simulink model "DC_grid_simple"  (R2018a)
settings: Solver=VariableStepAuto  StartTime=0.0  StopTime=10  RelTol=1e-3
values from neighbouring files (symbols this model uses):
  inputsFromWS = Simulink.Parameter(inputArray)    [DC_grid.m]    (also in QlearningEMS.m; QlearningEMS_Average.m; init_for_DC_grid.m)
libraries: SignalEditorBlockLib x1, powerlib x1
settings Model: SimulationMode=accelerator  Creator=David Pasdeloup  LastModifiedBy=David Pasdeloup
settings DataIOCC: FinalStateName=myOperPoint  LoadInitialState=on  SaveFinalState=on  SaveCompleteFinalSimState=on
settings DebuggingCC: MaxConsecutiveZCsMsg=none

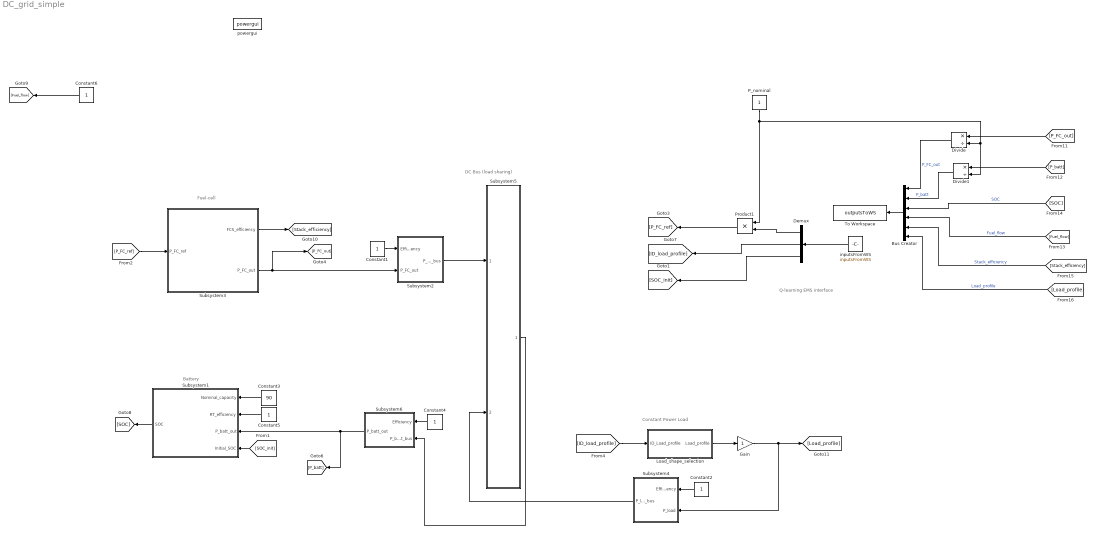
== system DC_grid_simple ==
  note: DC Bus (load sharing)
  note: Q-learning EMS interface
  note: Fuel-cell
  note: Battery
  note: Constant Power Load
  Bus Creator : BusCreator  Inputs=6
  Constant{1..2,4..6} (5 alike) : Constant
  Constant3 : Constant  Value=90
  Demux : Demux  Outputs=3
  Divide : Product  Inputs=*/
  Divide1 : Product  Inputs=*/
  Gain : Gain
  Load_shape_selection : Subsystem
  P_nominal : Constant
  Product1 : Product
  Subsystem1 : Subsystem
  Subsystem2 : Subsystem
  Subsystem3 : Subsystem
  Subsystem4 : Subsystem
  Subsystem5 : Subsystem
  Subsystem6 : Subsystem
  To Workspace : ToWorkspace  VariableName=outputsToWS  SaveFormat=Timeseries  SampleTime=-1
  inputsFromWS : Constant  Value=inputsFromWS
  powergui : powerlib/powergui  SimulationMode=Continuous  SampleTime=1e-6  frequency=60  Iterations=50  frequencyindice=0  Pbase=100e6  ErrMax=1e-4  UnitsV=kV  UnitsW=MW  buscounter=0  FunctionMessages=off  echomessages=off  EnableUseOfTLC=off  CurrentSourceSwitches=off  DisableSnubberDevices=off  DisableRonSwitches=off  DisableVfSwitches=off  DisplayEquations=off  SolverType=Tustin/Backward Euler (TBE)  Interpol=off  ExternalGateDelay=off  methode=off  Ts=100  x0status=blocks  SPID=on  SwTol=0  HookPort=off  RestoreLinks=warning  ResistiveCurrentMeasurement=off  Frange=[0:2:500]  Ylog=off  Xlog=on  ShowGrid=off  save=off  variable=ZData  structure=0  ZoomFFT=on  StartTime=0.0  cycles=1  DisplayStyle=1  fundamental=60  FreqAxis=off  MaxFrequency=1000  frequencyindicesteady=1  RmsSteady=1  display=off
  wires:
  Demux/1 -> Product1/2
  Demux/2 -> [ID_load_profile]
  Bus Creator/1 -> To Workspace/1
  [P_batt] -> Divide1/1
  Divide1/1 -> Bus Creator/2  "P_batt"
  inputsFromWS/1 -> Demux/1
  Product1/1 -> [P_FC_ref]
  Divide/1 -> Bus Creator/1  "P_FC_out"
  P_nominal/1 -> Divide1/2, Divide/2, Product1/1
  [P_FC_out] -> Divide/1
  [SOC] -> Bus Creator/3  "SOC"
  [Fuel_flow] -> Bus Creator/4  "Fuel_flow"
  [Stack_efficiency] -> Bus Creator/5  "Stack_efficiency"
  [ID_load_profile] -> Load_shape_selection/1(ID_Load_profile)
  Load_shape_selection/1(Load_profile) -> Gain/1
  [Load_profile] -> Bus Creator/6  "Load_profile"
  Demux/3 -> [SOC_init]
  Subsystem6/1(P_batt_out) -> [P_batt], Subsystem1/3(P_batt_out)
  Constant4/1 -> Subsystem6/1(Efficiency)
  Constant3/1 -> Subsystem1/1(Nominal_capacity)
  Constant5/1 -> Subsystem1/2(RT_efficiency)
  [SOC_init] -> Subsystem1/4(Initial_SOC)
  Subsystem1/1(SOC) -> [SOC]
  Constant1/1 -> Subsystem2/1(Efficiency)
  Subsystem3/2(P_FC_out) -> [P_FC_out], Subsystem2/2(P_FC_out)
  [P_FC_ref] -> Subsystem3/1(P_FC_ref)
  Subsystem3/1(FCS_efficiency) -> [Stack_efficiency]
  Constant2/1 -> Subsystem4/1(Efficiency)
  Subsystem2/1(P_FC_bus) -> Subsystem5/1(P_FC_bus)
  Subsystem4/1(P_load_bus) -> Subsystem5/2(P_load_bus)
  Subsystem5/1(P_batt_bus) -> Subsystem6/2(P_batt_bus)
  Constant6/1 -> [Fuel_flow]
  Gain/1 -> Subsystem4/2(P_load), [Load_profile]

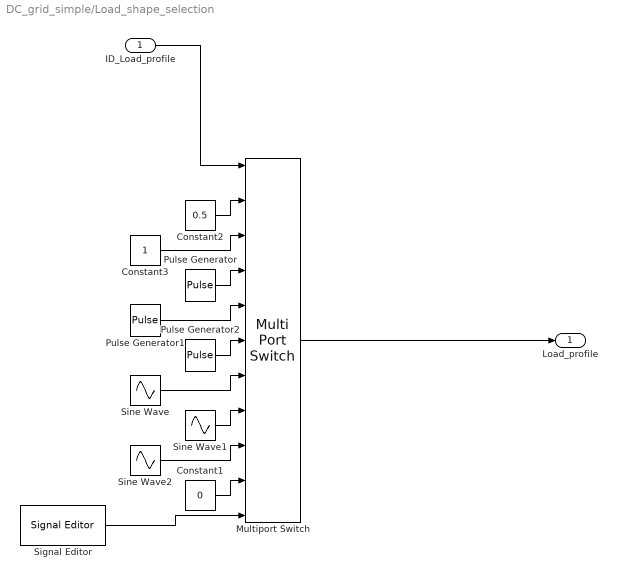
== system DC_grid_simple/Load_shape_selection ==
  ID_Load_profile : Inport
  Constant1 : Constant  Value=0
  Constant2 : Constant  Value=0.5
  Constant3 : Constant
  Multiport Switch : MultiPortSwitch  DataPortOrder=Specify indices  DataPortIndices={1,2,3,4,5,6,7,8,9,10}
  Pulse Generator : DiscretePulseGenerator  PulseType=Time based  Period=1  PulseWidth=50  PhaseDelay=10
  Pulse Generator1 : DiscretePulseGenerator  PulseType=Time based  Period=5  PulseWidth=50  PhaseDelay=10
  Pulse Generator2 : DiscretePulseGenerator  PulseType=Time based  Period=60  PulseWidth=50  PhaseDelay=10
  Signal Editor : SignalEditorBlockLib/Signal Editor  FileName=myLoadSample.mat  ActiveScenario=myLoadSample  ActiveSignal=mySample  IsBus=off  OutputBusObjectStr=Bus: BusObject  SampleTime=0  Interpolate=off  ZeroCross=off  OutputAfterFinalValue=Setting to zero  Unit=inherit
  Sine Wave : Sin  Amplitude=0.5  Bias=0.5  Frequency=2*pi  Phase=-pi/2  SampleTime=0
  Sine Wave1 : Sin  Amplitude=0.5  Bias=0.5  Frequency=2*pi/5  Phase=-pi/2  SampleTime=0
  Sine Wave2 : Sin  Amplitude=0.5  Bias=0.5  Frequency=2*pi/60  Phase=-pi/2  SampleTime=0
  Load_profile : Outport
  wires:
  Constant1/1 -> Multiport Switch/10
  Sine Wave2/1 -> Multiport Switch/9
  Pulse Generator2/1 -> Multiport Switch/6
  Sine Wave/1 -> Multiport Switch/7
  Constant2/1 -> Multiport Switch/2
  Constant3/1 -> Multiport Switch/3
  Pulse Generator1/1 -> Multiport Switch/5
  Pulse Generator/1 -> Multiport Switch/4
  Sine Wave1/1 -> Multiport Switch/8
  Multiport Switch/1 -> Load_profile/1
  ID_Load_profile/1 -> Multiport Switch/1
  Signal Editor/1 -> Multiport Switch/11

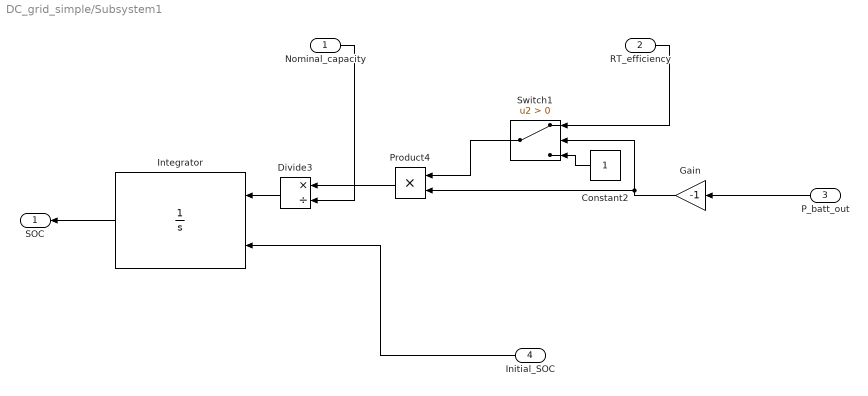
== system DC_grid_simple/Subsystem1 ==
  Nominal_capacity : Inport
  RT_efficiency : Inport  Port=2
  P_batt_out : Inport  Port=3
  Initial_SOC : Inport  Port=4
  Constant2 : Constant
  Divide3 : Product  Inputs=*/
  Gain : Gain  Gain=-1
  Integrator : Integrator  InitialConditionSource=external  LimitOutput=on  UpperSaturationLimit=1  LowerSaturationLimit=0
  Product4 : Product
  Switch1 : Switch  Criteria=u2 > Threshold
  SOC : Outport
  wires:
  Nominal_capacity/1 -> Divide3/2
  Constant2/1 -> Switch1/3
  Gain/1 -> Product4/2, Switch1/2
  Initial_SOC/1 -> Integrator/2
  RT_efficiency/1 -> Switch1/1
  Switch1/1 -> Product4/1
  Product4/1 -> Divide3/1
  Divide3/1 -> Integrator/1
  Integrator/1 -> SOC/1
  P_batt_out/1 -> Gain/1

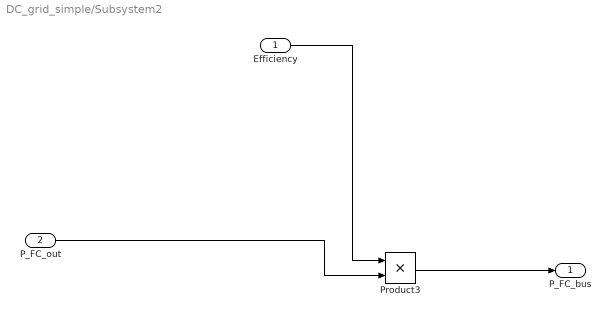
== system DC_grid_simple/Subsystem2 ==
  Efficiency : Inport
  P_FC_out : Inport  Port=2
  Product3 : Product
  P_FC_bus : Outport
  wires:
  P_FC_out/1 -> Product3/2
  Efficiency/1 -> Product3/1
  Product3/1 -> P_FC_bus/1

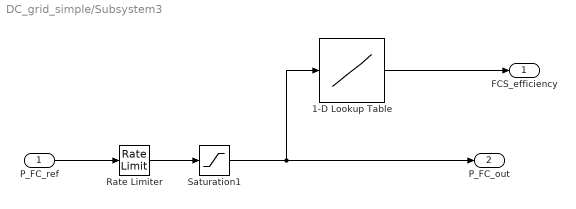
== system DC_grid_simple/Subsystem3 ==
  P_FC_ref : Inport
  1-D Lookup Table : Lookup_n-D  NumberOfTableDimensions=1  BreakpointsForDimension1=[0.000 0.025 0.050 0.075 0.100 0.125 0.150 0.175 0.200 0.225 0.250 0.275 0.300 0.325 0.350 0.375 0.400 0.425 0.450 0.475 0.500 0.525 0.550 0.575 0.600 0.625 0.650 0.675 0.700 0.725 0.750 0.775 0.800 0.825 0.850 0.875 0.900 0.925 0.950 0.975 1.000 ]  BreakpointsForDimension1FirstPoint=0  BreakpointsForDimension1Spacing=0.05  Table=[0.000 21.539 37.437 48.565 55.795 60.000 62.052 62.822 63.165 63.495 63.787 64.000 64.100 64.095 64.000 63.832 63.602 63.321 63.000 62.649 62.271 61.868 61.444 61.000 60.537 60.050 59.531 58.974 58.371 57.715 57.000 56.218 55.362 54.424 53.399 52.278 51.056 49.723 48.275 46.703 45.000 ]  InterpMethod=Cubic spline  ExtrapMethod=Cubic spline  InternalRulePriority=Speed  RndMeth=Simplest  InputSameDT=on
  Rate Limiter : RateLimiter  RisingSlewLimit=0.0769  FallingSlewLimit=-0.0769  SampleTimeMode=inherited
  Saturation1 : Saturate  UpperLimit=1  LowerLimit=0.1
  FCS_efficiency : Outport
  P_FC_out : Outport  Port=2
  wires:
  Saturation1/1 -> 1-D Lookup Table/1, P_FC_out/1
  Rate Limiter/1 -> Saturation1/1
  P_FC_ref/1 -> Rate Limiter/1
  1-D Lookup Table/1 -> FCS_efficiency/1

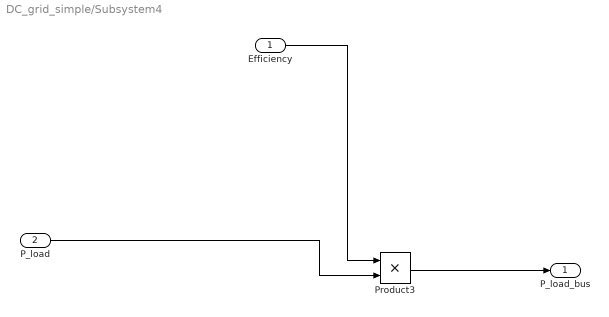
== system DC_grid_simple/Subsystem4 ==
  Efficiency : Inport
  P_load : Inport  Port=2
  Product3 : Product
  P_load_bus : Outport
  wires:
  P_load/1 -> Product3/2
  Efficiency/1 -> Product3/1
  Product3/1 -> P_load_bus/1

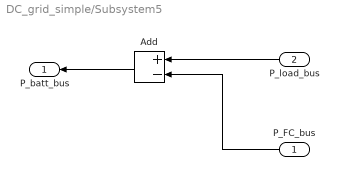
== system DC_grid_simple/Subsystem5 ==
  P_FC_bus : Inport
  P_load_bus : Inport  Port=2
  Add : Sum  Inputs=+-
  P_batt_bus : Outport
  wires:
  P_FC_bus/1 -> Add/2
  P_load_bus/1 -> Add/1
  Add/1 -> P_batt_bus/1

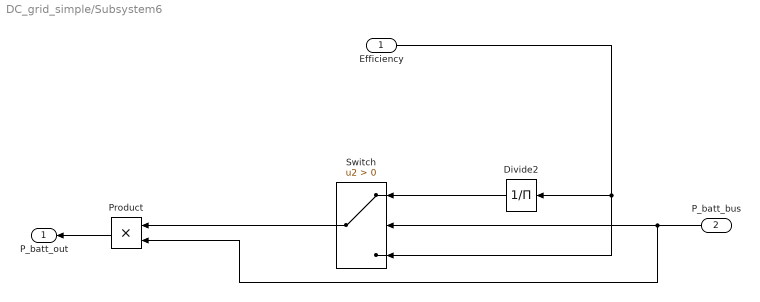
== system DC_grid_simple/Subsystem6 ==
  Efficiency : Inport
  P_batt_bus : Inport  Port=2
  Divide2 : Product  Inputs=/
  Product : Product
  Switch : Switch  Criteria=u2 > Threshold
  P_batt_out : Outport
  wires:
  Divide2/1 -> Switch/1
  Efficiency/1 -> Divide2/1, Switch/3
  P_batt_bus/1 -> Product/2, Switch/2
  Product/1 -> P_batt_out/1
  Switch/1 -> Product/1
